simulink model "IM_Close_Loop"  (R2019b)
settings: Solver=VariableStepAuto  StartTime=0.0  StopTime=70  RelTol=1e-3
values from neighbouring files (symbols this model uses):
  B = 0.068    [IM_Model_Parameters.m]
  fn = 50    [IM_Model_Parameters.m]
  J = 0.4    [IM_Model_Parameters.m]
  k = 0.009    [IM_Model_Parameters.m]
  Lks = Ls - Lm^2/Lr    (= 0.00442538071066)    [IM_Model_Parameters.m]
  Lm = 57e-3    (= 0.057)    [IM_Model_Parameters.m]
  np = 3    [IM_Model_Parameters.m]
  r = 4    [IM_Model_Parameters.m]
  R_ix = pidtune(G_ix, "PI", bw_ix, opts)    [IM_Model_Parameters.m]
  R_rFlx = pidtune(G_rFlx, "PI", bw_rFlx, opts)    [IM_Model_Parameters.m]
  R_spd = pidtune(G_spd, "PI", bw_spd, opts)    [IM_Model_Parameters.m]
  Rr = 0.175    [IM_Model_Parameters.m]
  Rs = 0.24    [IM_Model_Parameters.m]
  vsat = 380    [IM_Model_Parameters.m]
  wb = 2*pi*fn/np    (= 104.71975512)    [IM_Model_Parameters.m]
undefined symbols (not defined in the file or in its folder): sigbuilder_block
libraries: simulink x4
settings Model: Creator=hassancurrimbhoy  LastModifiedBy=hassancurrimbhoy
settings SolverCC: ZeroCrossAlgorithm=Adaptive
settings DebuggingCC: IgnoredZcDiagnostic=none

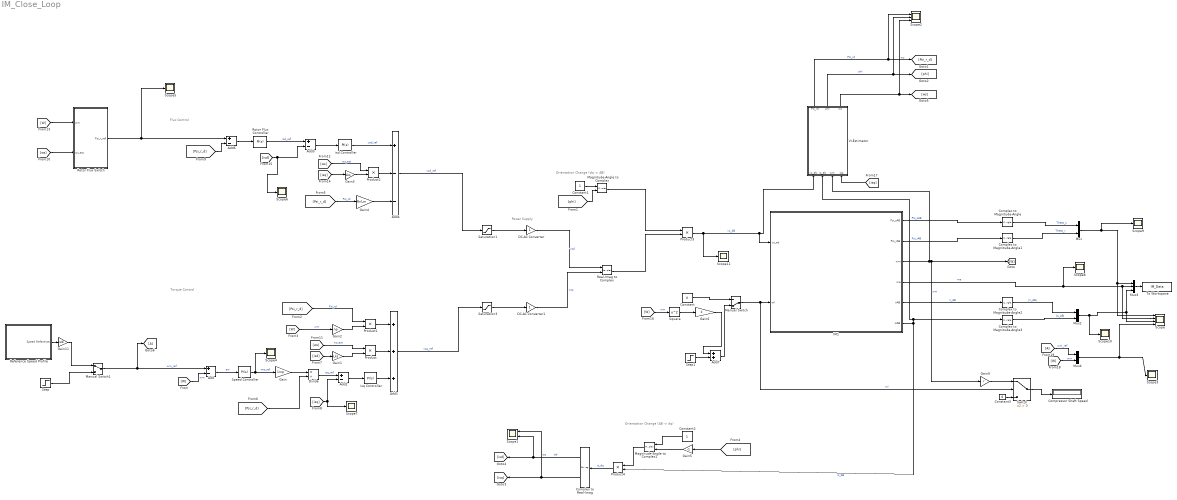
== system IM_Close_Loop ==
  note: Orientation Change (AB -> dq)
  note: Orientation Change (dq -> AB)
  note: Torque Control
  note: Flux Control
  note: Power Supply
  Add{,2..3,6} (4 alike) : Sum  Inputs=+-
  Add1 : Sum  Inputs=+++
  Add4 : Sum  Inputs=+--
  Add7 : Sum
  Complex to Magnitude-Angle : ComplexToMagnitudeAngle  Output=Angle
  Complex to Magnitude-Angle1 : ComplexToMagnitudeAngle  Output=Angle
  Complex to Magnitude-Angle2 : ComplexToMagnitudeAngle  Output=Magnitude
  Complex to Magnitude-Angle3 : ComplexToMagnitudeAngle  Output=Magnitude
  Complex to Real-Imag : ComplexToRealImag
  Compressor Shaft Speed : Display
  Constant : Constant  Value=0
  Constant1 : Constant
  Constant2 : Constant
  Constant3 : Constant  Value=0
  DC-AC Converter : Gain
  DC-AC Converter1 : Gain
  Divide : Product  Inputs=*/
  Gain : Gain  Gain=1/np
  Gain1 : Gain  Gain=Lks
  Gain11 : Gain  Gain=wb
  Gain2 : Gain  Gain=np
  Gain3 : Gain  Gain=Lks
  Gain4 : Gain  Gain=Rr/Lm
  Gain5 : Gain  Gain=-1
  Gain6 : Gain  Gain=k
  Gain9 : Gain  Gain=r
  IM1 : Subsystem
      mask Display: image('$imagefile'); % Use "Edit Image" on toolstrip to change.
  Magnitude-Angle to Complex : MagnitudeAngleToComplex
  Magnitude-Angle to Complex1 : MagnitudeAngleToComplex
  Manual Switch : ManualSwitch  CurrentSetting=0
  Manual Switch1 : ManualSwitch
  Mux : Mux  Inputs=2
  Mux2 : Mux  Inputs=2
  Mux3 : Mux  Inputs=3
  Mux4 : Mux  Inputs=2
  Product{,1..4} (5 alike) : Product
  Real-Imag to Complex : RealImagToComplex
  Reference Speed Profile : Subsystem  Tag=STV Subsys  LoadFcn=sigbuilder_block('load');  StartFcn=sigbuilder_block('start');  StopFcn=sigbuilder_block('stop');  ClipboardFcn=sigbuilder_block('clipboard');  mask(Sigbuilder block){tuvar=[0:10]}
      mask help: Simulink:masks:SigbuilderBlock_MD
      mask init:
      | if ~strcmp(get_param(bdroot(gcbh),'SimulationStatus'),'stopped') tuvar = sigbuilder_block('maskInit'); end
      settings: CopyFcn=sigbuilder_block('copy');  DeleteFcn=sigbuilder_block('delete');  ModelCloseFcn=sigbuilder_block('modelClose');  PreSaveFcn=sigbuilder_block('preSave');  PauseFcn=sigbuilder_block('pause');  ContinueFcn=sigbuilder_block('continue');  NameChangeFcn=sigbuilder_block('namechange');  OpenFcn=sigbuilder_block('open',[437.6 199.2 550.4 400 ]);  CloseFcn=sigbuilder_block('close');
      mask Display: plot(0, 0, 100, 100,[2, 2, 32, 32, 2], [68, 8, 8, 68, 68],[32, 2], [38, 38], [32, 19, 2],[53, 60, 44], [32, 17, 17, 2],[16, 16, 31, 31]);txt = getActiveGroup(gcbh);text(2, 100, txt,'verticalAlignment', 'top');
  Rotor Flux Controller : simulink/Continuous/PID Controller  Controller=PI  Form=Parallel  TimeDomain=Continuous-time  SampleTime=-1  IntegratorMethod=Forward Euler  FilterMethod=Forward Euler  ControllerParametersSource=internal  P=R_rFlx.Kp  I=R_rFlx.Ki  D=0  UseFilter=on  N=100  TunerSelectOption=Transfer Function Based (PID Tuner App)  InitialConditionSource=internal  InitialConditionForIntegrator=0  InitialConditionForFilter=0  DifferentiatorICPrevScaledInput=0  ExternalReset=none  TrackingMode=off  Kt=1  LimitOutput=off  UpperSaturationLimit=inf  LowerSaturationLimit=-inf  LinearizeAsGain=on  AntiWindupMode=none  Kb=1  POutMin=[]  POutMax=[]  IOutMin=[]  IOutMax=[]  DOutMin=[]  DOutMax=[]  NOutMin=[]  NOutMax=[]  SumOutMin=[]  SumOutMax=[]  SaturationOutMin=[]  SaturationOutMax=[]  PParamMin=[]  PParamMax=[]  IParamMin=[]  IParamMax=[]  DParamMin=[]  DParamMax=[]  NParamMin=[]  NParamMax=[]  KbParamMin=[]  KbParamMax=[]  KtParamMin=[]  KtParamMax=[]  KbOutMin=[]  KbOutMax=[]  KtOutMin=[]  KtOutMax=[]  IntegratorOutMin=[]  IntegratorOutMax=[]  FilterOutMin=[]  FilterOutMax=[]  SumI1OutMin=[]  SumI1OutMax=[]  SumI2OutMin=[]  SumI2OutMax=[]  SumI3OutMin=[]  SumI3OutMax=[]  SumI4OutMin=[]  SumI4OutMax=[]  SumDOutMin=[]  SumDOutMax=[]  DifferentiatorOutMin=[]  DifferentiatorOutMax=[]  FilterDiffOutCoefMin=[]  FilterDiffOutCoefMax=[]  ReciprocalOutMin=[]  ReciprocalOutMax=[]  SumDenOutMin=[]  SumDenOutMax=[]  SumNumOutMin=[]  SumNumOutMax=[]  DivideOutMin=[]  DivideOutMax=[]  IntegratorContinuousStateAttributes=''  IntegratorStateMustResolveToSignalObject=off  IntegratorRTWStateStorageClass=Auto  FilterContinuousStateAttributes=''  FilterStateMustResolveToSignalObject=off  FilterRTWStateStorageClass=Auto  ParallelPVariant=InternalParameters  IdealPVariant=Disabled  IVariant=InternalParameters  DVariant=Disabled  IntegratorVariant=Continuous  SatVariant=Disabled  AWVariant=Passthrough  PCopyVariant=Disabled  TRVariant=Disabled  FdbkBlocksVariant=Forward  IdealPFdbkVariant=Disabled  SatFdbkVariant=Disabled  DerivativeFilterVariant=Disabled  NVariant=Disabled  NCopyVariant=Disabled_SignalSpec  FilterICVariant=Disabled  IntegratorICVariant=InternalICs  ExternalResetVariant=Disabled  TRSumVariant=Passthrough  SumFdbkVariant=Disabled  SumVariant=Sum_PI
  Rotor Flux Switch : Subsystem
  Saturation1 : Saturate  UpperLimit=vsat  LowerLimit=-vsat  LinearizeAsGain=off  ZeroCross=off
  Saturation3 : Saturate  UpperLimit=vsat  LowerLimit=-vsat  LinearizeAsGain=off  ZeroCross=off
  Scope : Scope  NumInputPorts=4
  Scope1 : Scope  NumInputPorts=2
  Scope{3..11} (9 alike) : Scope
  Scope2 : Scope  NumInputPorts=3
  Speed Controller : simulink/Continuous/PID Controller  Controller=PI  Form=Parallel  TimeDomain=Continuous-time  SampleTime=-1  IntegratorMethod=Forward Euler  FilterMethod=Forward Euler  ControllerParametersSource=internal  P=R_spd.Kp  I=R_spd.Ki  D=0  UseFilter=on  N=100  TunerSelectOption=Transfer Function Based (PID Tuner App)  InitialConditionSource=internal  InitialConditionForIntegrator=0  InitialConditionForFilter=0  DifferentiatorICPrevScaledInput=0  ExternalReset=none  TrackingMode=off  Kt=1  LimitOutput=off  UpperSaturationLimit=inf  LowerSaturationLimit=-inf  LinearizeAsGain=on  AntiWindupMode=none  Kb=1  POutMin=[]  POutMax=[]  IOutMin=[]  IOutMax=[]  DOutMin=[]  DOutMax=[]  NOutMin=[]  NOutMax=[]  SumOutMin=[]  SumOutMax=[]  SaturationOutMin=[]  SaturationOutMax=[]  PParamMin=[]  PParamMax=[]  IParamMin=[]  IParamMax=[]  DParamMin=[]  DParamMax=[]  NParamMin=[]  NParamMax=[]  KbParamMin=[]  KbParamMax=[]  KtParamMin=[]  KtParamMax=[]  KbOutMin=[]  KbOutMax=[]  KtOutMin=[]  KtOutMax=[]  IntegratorOutMin=[]  IntegratorOutMax=[]  FilterOutMin=[]  FilterOutMax=[]  SumI1OutMin=[]  SumI1OutMax=[]  SumI2OutMin=[]  SumI2OutMax=[]  SumI3OutMin=[]  SumI3OutMax=[]  SumI4OutMin=[]  SumI4OutMax=[]  SumDOutMin=[]  SumDOutMax=[]  DifferentiatorOutMin=[]  DifferentiatorOutMax=[]  FilterDiffOutCoefMin=[]  FilterDiffOutCoefMax=[]  ReciprocalOutMin=[]  ReciprocalOutMax=[]  SumDenOutMin=[]  SumDenOutMax=[]  SumNumOutMin=[]  SumNumOutMax=[]  DivideOutMin=[]  DivideOutMax=[]  IntegratorContinuousStateAttributes=''  IntegratorStateMustResolveToSignalObject=off  IntegratorRTWStateStorageClass=Auto  FilterContinuousStateAttributes=''  FilterStateMustResolveToSignalObject=off  FilterRTWStateStorageClass=Auto  ParallelPVariant=InternalParameters  IdealPVariant=Disabled  IVariant=InternalParameters  DVariant=Disabled  IntegratorVariant=Continuous  SatVariant=Disabled  AWVariant=Passthrough  PCopyVariant=Disabled  TRVariant=Disabled  FdbkBlocksVariant=Forward  IdealPFdbkVariant=Disabled  SatFdbkVariant=Disabled  DerivativeFilterVariant=Disabled  NVariant=Disabled  NCopyVariant=Disabled_SignalSpec  FilterICVariant=Disabled  IntegratorICVariant=InternalICs  ExternalResetVariant=Disabled  TRSumVariant=Passthrough  SumFdbkVariant=Disabled  SumVariant=Sum_PI
  Square : Math  Operator=square  SignedPower=off  SaturateOnIntegerOverflow=on
  Step : Step  Time=0.1  After=wb  SampleTime=0
  Step1 : Step  Time=55  After=5  SampleTime=0
  Switch : Switch  Criteria=u2 > Threshold
  To Workspace : ToWorkspace  VariableName=IM_Data  SaveFormat=Timeseries  SampleTime=-1
  VI-Estimator : Subsystem
  isd Controller : simulink/Continuous/PID Controller  Controller=PI  Form=Parallel  TimeDomain=Continuous-time  SampleTime=-1  IntegratorMethod=Forward Euler  FilterMethod=Forward Euler  ControllerParametersSource=internal  P=R_ix.Kp  I=R_ix.Ki  D=0  UseFilter=on  N=100  TunerSelectOption=Transfer Function Based (PID Tuner App)  InitialConditionSource=internal  InitialConditionForIntegrator=0  InitialConditionForFilter=0  DifferentiatorICPrevScaledInput=0  ExternalReset=none  TrackingMode=off  Kt=1  LimitOutput=off  UpperSaturationLimit=inf  LowerSaturationLimit=-inf  LinearizeAsGain=on  AntiWindupMode=none  Kb=1  POutMin=[]  POutMax=[]  IOutMin=[]  IOutMax=[]  DOutMin=[]  DOutMax=[]  NOutMin=[]  NOutMax=[]  SumOutMin=[]  SumOutMax=[]  SaturationOutMin=[]  SaturationOutMax=[]  PParamMin=[]  PParamMax=[]  IParamMin=[]  IParamMax=[]  DParamMin=[]  DParamMax=[]  NParamMin=[]  NParamMax=[]  KbParamMin=[]  KbParamMax=[]  KtParamMin=[]  KtParamMax=[]  KbOutMin=[]  KbOutMax=[]  KtOutMin=[]  KtOutMax=[]  IntegratorOutMin=[]  IntegratorOutMax=[]  FilterOutMin=[]  FilterOutMax=[]  SumI1OutMin=[]  SumI1OutMax=[]  SumI2OutMin=[]  SumI2OutMax=[]  SumI3OutMin=[]  SumI3OutMax=[]  SumI4OutMin=[]  SumI4OutMax=[]  SumDOutMin=[]  SumDOutMax=[]  DifferentiatorOutMin=[]  DifferentiatorOutMax=[]  FilterDiffOutCoefMin=[]  FilterDiffOutCoefMax=[]  ReciprocalOutMin=[]  ReciprocalOutMax=[]  SumDenOutMin=[]  SumDenOutMax=[]  SumNumOutMin=[]  SumNumOutMax=[]  DivideOutMin=[]  DivideOutMax=[]  IntegratorContinuousStateAttributes=''  IntegratorStateMustResolveToSignalObject=off  IntegratorRTWStateStorageClass=Auto  FilterContinuousStateAttributes=''  FilterStateMustResolveToSignalObject=off  FilterRTWStateStorageClass=Auto  ParallelPVariant=InternalParameters  IdealPVariant=Disabled  IVariant=InternalParameters  DVariant=Disabled  IntegratorVariant=Continuous  SatVariant=Disabled  AWVariant=Passthrough  PCopyVariant=Disabled  TRVariant=Disabled  FdbkBlocksVariant=Forward  IdealPFdbkVariant=Disabled  SatFdbkVariant=Disabled  DerivativeFilterVariant=Disabled  NVariant=Disabled  NCopyVariant=Disabled_SignalSpec  FilterICVariant=Disabled  IntegratorICVariant=InternalICs  ExternalResetVariant=Disabled  TRSumVariant=Passthrough  SumFdbkVariant=Disabled  SumVariant=Sum_PI
  isq Controller : simulink/Continuous/PID Controller  Controller=PI  Form=Parallel  TimeDomain=Continuous-time  SampleTime=-1  IntegratorMethod=Forward Euler  FilterMethod=Forward Euler  ControllerParametersSource=internal  P=R_ix.Kp  I=R_ix.Ki  D=0  UseFilter=on  N=100  TunerSelectOption=Transfer Function Based (PID Tuner App)  InitialConditionSource=internal  InitialConditionForIntegrator=0  InitialConditionForFilter=0  DifferentiatorICPrevScaledInput=0  ExternalReset=none  TrackingMode=off  Kt=1  LimitOutput=off  UpperSaturationLimit=inf  LowerSaturationLimit=-inf  LinearizeAsGain=on  AntiWindupMode=none  Kb=1  POutMin=[]  POutMax=[]  IOutMin=[]  IOutMax=[]  DOutMin=[]  DOutMax=[]  NOutMin=[]  NOutMax=[]  SumOutMin=[]  SumOutMax=[]  SaturationOutMin=[]  SaturationOutMax=[]  PParamMin=[]  PParamMax=[]  IParamMin=[]  IParamMax=[]  DParamMin=[]  DParamMax=[]  NParamMin=[]  NParamMax=[]  KbParamMin=[]  KbParamMax=[]  KtParamMin=[]  KtParamMax=[]  KbOutMin=[]  KbOutMax=[]  KtOutMin=[]  KtOutMax=[]  IntegratorOutMin=[]  IntegratorOutMax=[]  FilterOutMin=[]  FilterOutMax=[]  SumI1OutMin=[]  SumI1OutMax=[]  SumI2OutMin=[]  SumI2OutMax=[]  SumI3OutMin=[]  SumI3OutMax=[]  SumI4OutMin=[]  SumI4OutMax=[]  SumDOutMin=[]  SumDOutMax=[]  DifferentiatorOutMin=[]  DifferentiatorOutMax=[]  FilterDiffOutCoefMin=[]  FilterDiffOutCoefMax=[]  ReciprocalOutMin=[]  ReciprocalOutMax=[]  SumDenOutMin=[]  SumDenOutMax=[]  SumNumOutMin=[]  SumNumOutMax=[]  DivideOutMin=[]  DivideOutMax=[]  IntegratorContinuousStateAttributes=''  IntegratorStateMustResolveToSignalObject=off  IntegratorRTWStateStorageClass=Auto  FilterContinuousStateAttributes=''  FilterStateMustResolveToSignalObject=off  FilterRTWStateStorageClass=Auto  ParallelPVariant=InternalParameters  IdealPVariant=Disabled  IVariant=InternalParameters  DVariant=Disabled  IntegratorVariant=Continuous  SatVariant=Disabled  AWVariant=Passthrough  PCopyVariant=Disabled  TRVariant=Disabled  FdbkBlocksVariant=Forward  IdealPFdbkVariant=Disabled  SatFdbkVariant=Disabled  DerivativeFilterVariant=Disabled  NVariant=Disabled  NCopyVariant=Disabled_SignalSpec  FilterICVariant=Disabled  IntegratorICVariant=InternalICs  ExternalResetVariant=Disabled  TRSumVariant=Passthrough  SumFdbkVariant=Disabled  SumVariant=Sum_PI
  wires:
  Add/1 -> Speed Controller/1  "ew"
  Speed Controller/1 -> Scope4/1, Gain/1  "me_ref"
  Gain/1 -> Divide/1
  Divide/1 -> Add2/1  "isq_ref"
  Product/1 -> Add1/2
  Gain1/1 -> Product/2
  [ws] -> Product/1  "ws_est"
  [W] -> Gain2/1  "wm"
  [Psi_r_d] -> Product1/1  "Psi_rd"
  Gain2/1 -> Product1/2
  Product1/1 -> Add1/1
  Add1/1 -> Saturation3/1  "vsq_ref"
  DC-AC Converter/1 -> Real-Imag to Complex/1  "vsd"
  Rotor Flux Controller/1 -> Add3/1  "isd_ref"
  Add3/1 -> isd Controller/1
  isd Controller/1 -> Add4/1  "usd_ref"
  Add4/1 -> Saturation1/1  "vsd_ref"
  DC-AC Converter1/1 -> Real-Imag to Complex/2  "vsq"
  [ws] -> Product2/1  "ws_est"
  Gain3/1 -> Product2/2
  Product2/1 -> Add4/2
  Gain4/1 -> Add4/3
  [W] -> Add/2  "wm"
  Magnitude-Angle to Complex/1 -> Product3/1
  VI-Estimator/2(phi) -> Scope2/2, [phi]  "phi"
  [phi] -> Magnitude-Angle to Complex/2
  Constant1/1 -> Magnitude-Angle to Complex/1
  Constant2/1 -> Magnitude-Angle to Complex1/1
  Magnitude-Angle to Complex1/1 -> Product4/1
  [phi] -> Gain5/1
  Gain5/1 -> Magnitude-Angle to Complex1/2
  Product4/1 -> Complex to Real-Imag/1  "is_dq"
  Complex to Real-Imag/1 -> Scope1/2, [isd]  "isd"
  Complex to Real-Imag/2 -> Scope1/1, [isq]  "isq"
  [isq] -> Add2/2, Scope7/1
  [isd] -> Gain1/1
  Add6/1 -> Rotor Flux Controller/1
  IM1/1(Psi_sAB) -> Complex to Magnitude-Angle/1  "Psi_sAB"
  Rotor Flux Switch/1(Psi_r_ref) -> Scope5/1, Add6/1
  Manual Switch/1 -> Switch/2, IM1/2(ml)  "ml"
  Constant/1 -> Manual Switch/1
  Complex to Magnitude-Angle/1 -> Mux/1  "Theta_s"
  Complex to Magnitude-Angle1/1 -> Mux/2  "Theta_r"
  Complex to Magnitude-Angle2/1 -> Mux2/1  "|ir_AB|"
  Complex to Magnitude-Angle3/1 -> Mux2/2  "|is_AB|"
  Mux/1 -> Scope9/1, Scope/1, Mux3/1
  Mux2/1 -> Scope10/1, Mux3/3, Scope/3
  Mux3/1 -> To Workspace/1
  Reference Speed Profile/1(Speed Reference) -> Gain11/1
  Step/1 -> Manual Switch1/2
  Manual Switch1/1 -> [A], Add/1  "wm_ref"
  Gain11/1 -> Manual Switch1/1
  [W] -> Mux4/2  "wm"
  [A] -> Mux4/1  "wm_ref"
  Mux4/1 -> Scope3/1, Scope/4
  [W] -> Square/1  "wm"
  Square/1 -> Gain6/1
  [isd] -> Scope6/1, Add3/2
  [isq] -> Gain3/1
  [W] -> Rotor Flux Switch/1(wm)
  [Psi_r_d] -> Gain4/1  "Psi_rd"
  [Psi_r_d] -> Add6/2
  Product3/1 -> Scope11/1, IM1/1(vs_ab), VI-Estimator/1(vs_ab)  "vs_AB"
  Real-Imag to Complex/1 -> Product3/2
  Add2/1 -> isq Controller/1
  isq Controller/1 -> Add1/3
  [Psi_r_d] -> Divide/2
  VI-Estimator/1(Psi_rd) -> Scope2/1, [Psi_r_d]  "Psi_rd"
  Saturation1/1 -> DC-AC Converter/1
  Saturation3/1 -> DC-AC Converter1/1
  [ws] -> Rotor Flux Switch/2(ws,est)
  IM1/2(Psi_rAB) -> Complex to Magnitude-Angle1/1  "Psi_rAB"
  IM1/3(wm) -> Gain9/1, [W], VI-Estimator/3(wm)  "wm"
  IM1/5(irAB) -> Complex to Magnitude-Angle2/1  "ir_AB"
  IM1/6(isAB) -> Complex to Magnitude-Angle3/1, VI-Estimator/2(is_ab), Product4/2  "is_AB"
  IM1/4(me) -> Scope8/1, Scope/2, Mux3/2  "me"
  Step1/1 -> Add7/2
  Gain6/1 -> Add7/1
  Add7/1 -> Manual Switch/2
  Switch/1 -> Compressor Shaft Speed/1
  Gain9/1 -> Switch/1
  Constant3/1 -> Switch/3
  VI-Estimator/3(ws) -> Scope2/3, [ws]  "ws"
  [isq] -> VI-Estimator/4(isq)

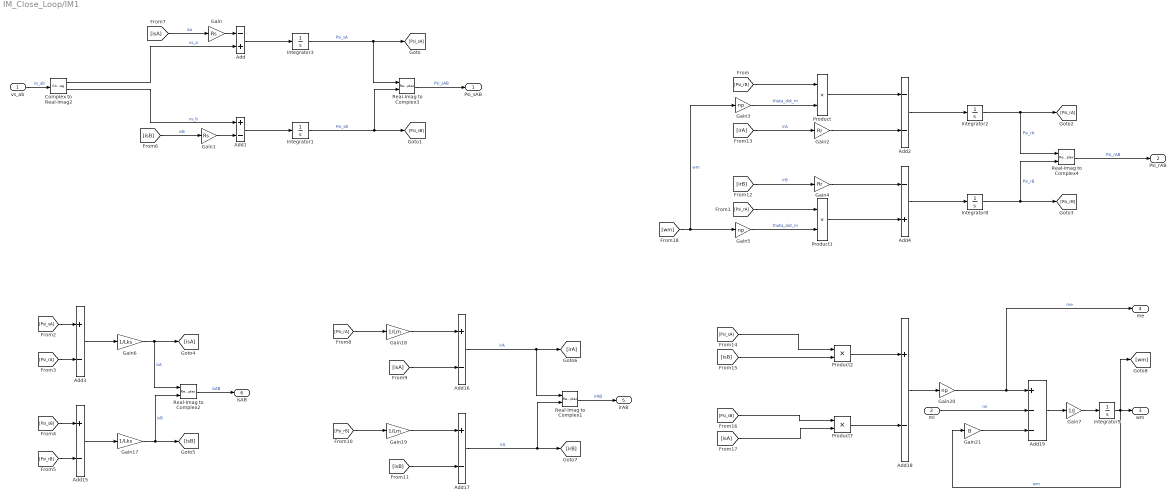
== system IM_Close_Loop/IM1 ==
  vs_ab : Inport
  ml : Inport  Port=2
  Add : Sum  Inputs=-+
  Add{1,3,15..18} (6 alike) : Sum  Inputs=+-
  Add19 : Sum  Inputs=+--
  Add2 : Sum  Inputs=--
  Add4 : Sum  Inputs=-+
  Complex to Real-Imag2 : ComplexToRealImag
  Gain : Gain  Gain=Rs
  Gain1 : Gain  Gain=Rs
  Gain17 : Gain  Gain=1/Lks
  Gain18 : Gain  Gain=1/Lm
  Gain19 : Gain  Gain=1/Lm
  Gain2 : Gain  Gain=Rr
  Gain20 : Gain  Gain=np
  Gain21 : Gain  Gain=B
  Gain3 : Gain  Gain=np
  Gain4 : Gain  Gain=Rr
  Gain5 : Gain  Gain=np
  Gain6 : Gain  Gain=1/Lks
  Gain7 : Gain  Gain=1/J
  Integrator{1..3,8..9} (5 alike) : Integrator
  Product{,1..2,7} (4 alike) : Product
  Real-Imag to Complex{1..4} (4 alike) : RealImagToComplex
  Psi_sAB : Outport
  Psi_rAB : Outport  Port=2
  wm : Outport  Port=3
  me : Outport  Port=4
  irAB : Outport  Port=5
  isAB : Outport  Port=6
  wires:
  vs_ab/1 -> Complex to Real-Imag2/1  "vs_ab"
  Complex to Real-Imag2/1 -> Add/2  "vs_a"
  Complex to Real-Imag2/2 -> Add1/1  "vs_b"
  [isA] -> Gain/1  "isa"
  Add/1 -> Integrator3/1
  Integrator3/1 -> [Psi_sA], Real-Imag to Complex3/1  "Psi_sA"
  Add1/1 -> Integrator1/1
  [isB] -> Gain1/1  "isB"
  Gain1/1 -> Add1/2
  Integrator1/1 -> Real-Imag to Complex3/2, [Psi_sB]  "Psi_sB"
  Integrator2/1 -> Real-Imag to Complex4/1, [Psi_rA]  "Psi_rA"
  Integrator8/1 -> [Psi_rB], Real-Imag to Complex4/2  "Psi_rB"
  Add2/1 -> Integrator2/1
  Add4/1 -> Integrator8/1
  Product/1 -> Add2/1
  Gain2/1 -> Add2/2
  [irA] -> Gain2/1  "irA"
  [Psi_rB] -> Product/1
  Gain3/1 -> Product/2  "theta_dot_m"
  Gain/1 -> Add/1
  Gain4/1 -> Add4/1
  [irB] -> Gain4/1  "irB"
  [wm] -> Gain3/1, Gain5/1  "wm"
  [Psi_rA] -> Product1/1
  Product1/1 -> Add4/2
  Gain5/1 -> Product1/2  "theta_dot_m"
  Add3/1 -> Gain6/1
  Gain6/1 -> Real-Imag to Complex2/1, [isA]  "isA"
  [Psi_sA] -> Add3/1
  [Psi_rA] -> Add3/2
  [Psi_rB] -> Add15/2
  Add15/1 -> Gain17/1
  [Psi_sB] -> Add15/1
  Gain17/1 -> Real-Imag to Complex2/2, [isB]  "isB"
  Add16/1 -> Real-Imag to Complex1/1, [irA]  "irA"
  Gain18/1 -> Add16/1
  [Psi_rA] -> Gain18/1
  [isA] -> Add16/2
  Add17/1 -> Real-Imag to Complex1/2, [irB]  "irA"
  Gain19/1 -> Add17/1
  [Psi_rB] -> Gain19/1
  [isB] -> Add17/2
  Gain20/1 -> me/1, Add19/1  "me"
  Product7/1 -> Add18/2
  Product2/1 -> Add18/1
  Gain21/1 -> Add19/3
  Add18/1 -> Gain20/1
  Integrator9/1 -> [wm], Gain21/1, wm/1  "wm"
  ml/1 -> Add19/2  "ml"
  [Psi_sA] -> Product2/1
  [isB] -> Product2/2
  [Psi_sB] -> Product7/1
  [isA] -> Product7/2
  Real-Imag to Complex1/1 -> irAB/1  "irAB"
  Real-Imag to Complex2/1 -> isAB/1  "isAB"
  Add19/1 -> Gain7/1
  Gain7/1 -> Integrator9/1
  Real-Imag to Complex4/1 -> Psi_rAB/1  "Psi_rAB"
  Real-Imag to Complex3/1 -> Psi_sAB/1  "Psi_sAB"

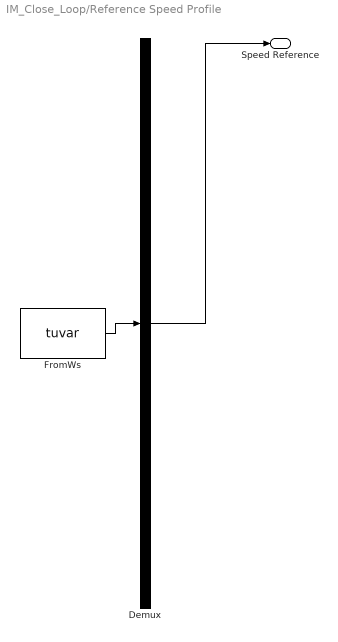
== system IM_Close_Loop/Reference Speed Profile ==
  Demux : Demux  Tag=STV Demux  Outputs=1
  FromWs : FromWorkspace  Tag=STV FromWs  VariableName=tuvar  SampleTime=0
      SigBuilderData=|
      | common.afterFinalStr = 'Extrapolate'
      | common.sampleTime = 0
      | dataSet.timeRange = [0 70]
      | dataSet.name = 'Group 1'
      | sbobj.Groups.Name = 'Group 1'
      | sbobj.Groups.Signals.Name = 'Speed Reference'
      | sbobj.Groups.Signals.XData = [0 20 30 40 60 70]
      | sbobj.Groups.Signals.YData = [0 0.1 0.1 0.2 0.2 0.2]
      | sbobj.Groups.TimeRange = [0 70]
  Speed Reference : Outport  Tag=STV Outport
  wires:
  Demux/1 -> Speed Reference/1
  FromWs/1 -> Demux/1

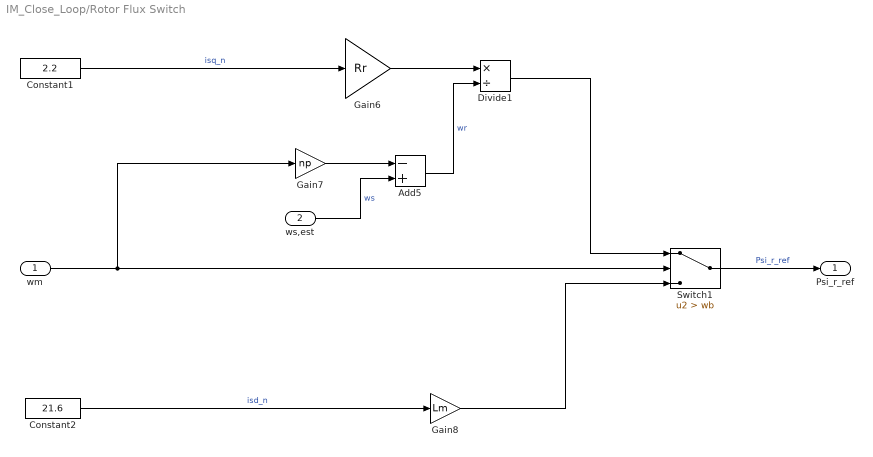
== system IM_Close_Loop/Rotor Flux Switch ==
  wm : Inport
  ws,est : Inport  Port=2
  Add5 : Sum  Inputs=-+
  Constant1 : Constant  Value=2.2
  Constant2 : Constant  Value=21.6
  Divide1 : Product  Inputs=*/
  Gain6 : Gain  Gain=Rr
  Gain7 : Gain  Gain=np
  Gain8 : Gain  Gain=Lm
  Switch1 : Switch  Criteria=u2 > Threshold  Threshold=wb
  Psi_r_ref : Outport
  wires:
  Constant2/1 -> Gain8/1  "isd_n"
  ws,est/1 -> Add5/2  "ws"
  Add5/1 -> Divide1/2  "wr"
  Switch1/1 -> Psi_r_ref/1  "Psi_r_ref"
  Gain8/1 -> Switch1/3
  Constant1/1 -> Gain6/1  "isq_n"
  Gain7/1 -> Add5/1
  Divide1/1 -> Switch1/1
  Gain6/1 -> Divide1/1
  wm/1 -> Switch1/2, Gain7/1

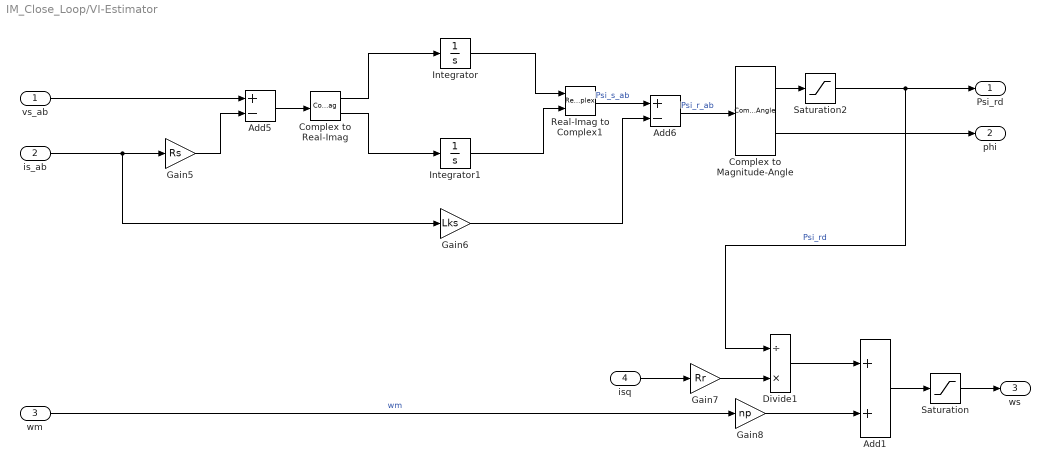
== system IM_Close_Loop/VI-Estimator ==
  vs_ab : Inport
  is_ab : Inport  Port=2
  wm : Inport  Port=3
  isq : Inport  Port=4
  Add1 : Sum
  Add5 : Sum  Inputs=+-
  Add6 : Sum  Inputs=+-
  Complex to Magnitude-Angle : ComplexToMagnitudeAngle
  Complex to Real-Imag : ComplexToRealImag
  Divide1 : Product  Inputs=/*
  Gain5 : Gain  Gain=Rs
  Gain6 : Gain  Gain=Lks
  Gain7 : Gain  Gain=Rr
  Gain8 : Gain  Gain=np
  Integrator : Integrator
  Integrator1 : Integrator
  Real-Imag to Complex1 : RealImagToComplex
  Saturation : Saturate  UpperLimit=2*pi*fn  LowerLimit=0
  Saturation2 : Saturate  UpperLimit=5  LowerLimit=0.1  LinearizeAsGain=off  ZeroCross=off
  Psi_rd : Outport
  phi : Outport  Port=2
  ws : Outport  Port=3
  wires:
  vs_ab/1 -> Add5/1
  Gain5/1 -> Add5/2
  Complex to Real-Imag/1 -> Integrator/1
  Complex to Real-Imag/2 -> Integrator1/1
  Add6/1 -> Complex to Magnitude-Angle/1  "Psi_r_ab"
  Gain6/1 -> Add6/2
  Integrator1/1 -> Real-Imag to Complex1/2
  Integrator/1 -> Real-Imag to Complex1/1
  Real-Imag to Complex1/1 -> Add6/1  "Psi_s_ab"
  Add5/1 -> Complex to Real-Imag/1
  is_ab/1 -> Gain6/1, Gain5/1
  Complex to Magnitude-Angle/2 -> phi/1
  Gain7/1 -> Divide1/2
  isq/1 -> Gain7/1
  Gain8/1 -> Add1/2
  Saturation/1 -> ws/1
  wm/1 -> Gain8/1  "wm"
  Divide1/1 -> Add1/1
  Add1/1 -> Saturation/1
  Complex to Magnitude-Angle/1 -> Saturation2/1
  Saturation2/1 -> Divide1/1, Psi_rd/1  "Psi_rd"
